simulink model "QuadcopterCompleteModel"  (R2015a)
settings: Solver=ode3  StartTime=0.0  StopTime=20  FixedStep=T_sim  RelTol=1e-5
values from neighbouring files (symbols this model uses):
  A_x = 0.015    [SetupComplete.m]
  A_y = A_x    (= 0.015)    [SetupComplete.m]
  A_z = 0.16    [SetupComplete.m]
  C_x = 1.2    [SetupComplete.m]
  C_y = C_x    (= 1.2)    [SetupComplete.m]
  C_z = 2.2    [SetupComplete.m]
  CG = [0,0,0.02]    [SetupComplete.m]
  I_BAC = diag( [Ix,Iy,Iz])    [SetupComplete.m]
  Initial_Omegas = Omega_hover*ones(4,1)    [Run4Copter.m]
  Initial_Torques = Torque_hover*ones(4,1)    [Run4Copter.m]
  k_quat = 100    [SetupComplete.m]
  l = 0.345    [SetupComplete.m]
  m = 3.51    [SetupComplete.m]
  M_eq = 0.001    [SetupComplete.m]
  R = 0.254    [SetupComplete.m]
  rho = 1.225    [SetupComplete.m]
  Rotation_sign = [ 1,-1,1,-1]    [SetupComplete.m]
  throtle_0 = 0.4    [Run4Copter.m]
undefined symbols (not defined in the file or in its folder): DOWN_0, EAST_0, NORTH_0, P_0, Q_0, R_0, U_0, V_0, W_0
libraries: MCopter x5, simulink_extras x1
settings Model: ExtModeTrigDuration=5000  Creator=alumno4  LastModifiedBy=David
settings SolverCC: PositivePriorityOrder=on
settings DataIOCC: ExternalInput=getinputstruct(op_trim1)  InitialState=getstatestruct(op_trim1)  SignalLoggingSaveFormat=ModelDataLogs
settings OptimizationCC: InlineParams=on  ExpressionDepthLimit=2147483647
settings DebuggingCC: UnderspecifiedInitializationDetection=Classic  MergeDetectMultiDrivingBlocksExec=none  SolverPrmCheckMsg=warning  FcnCallInpInsideContextMsg=UseLocalSettings  StateNameClashWarn=warning
settings RTWCC: SystemTargetFile=quarc_windows.tlc  TemplateMakefile=quarc_default_tmf  Description=QUARC Win32 Target
settings STFCustomTargetCC: TargetLibSuffix=.lib  TargetPreCompLibLocation=C:\PROGRA~2\QUARC\lib\2011a\windows\release  CodeReplacementLibrary=C89/C90 (ANSI)  GenerateSampleERTMain=off  GeneratePreprocessorConditionals=Disable all  ERTCustomFileBanners=off  SupportNonInlinedSFcns=on  SupportVariableSizeSignals=off  MATLABClassNameForMDSCustomization=Simulink.SoftwareTarget.GRTCustomization  CPPClassGenCompliant=on  GRTInterface=on  SystemTargetFile=quarc_windows.tlc
settings GRTTargetCC: TargetPreCompLibLocation=C:\PROGRA~2\QUARC\lib\2011a\windows\release  CodeReplacementLibrary=C89/C90 (ANSI)  ParMdlRefBuildCompliant=off  CompOptLevelCompliant=off  ConcurrentExecutionCompliant=off  CombineOutputUpdateFcns=off  MatFileLogging=off  GRTInterface=on  ExtMode=on  ExtModeMexFile=quarc_comm

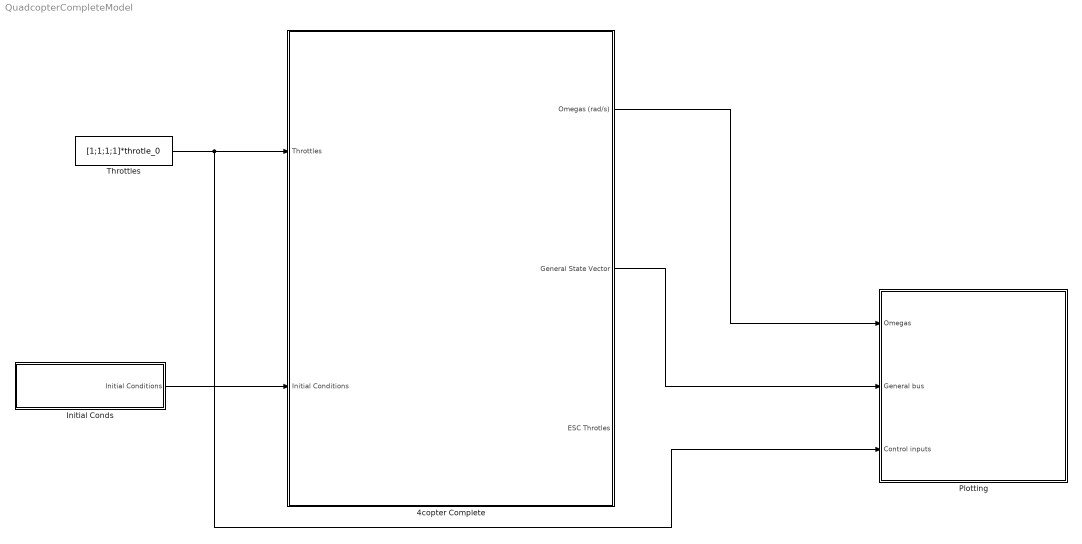
== system QuadcopterCompleteModel ==
  4copter Complete : Subsystem  TreatAsAtomicUnit=on
  Initial Conds : Subsystem  TreatAsAtomicUnit=on
  Plotting : Subsystem
  Throttles : Constant  Value=[1;1;1;1]*throtle_0
  wires:
  Initial Conds/1(Initial Conditions) -> 4copter Complete/2(Initial Conditions)
  Throttles/1 -> Plotting/3(Control inputs), 4copter Complete/1(Throttles)
  4copter Complete/1(Omegas (rad/s)) -> Plotting/1(Omegas)
  4copter Complete/2(General State Vector) -> Plotting/2(General bus)

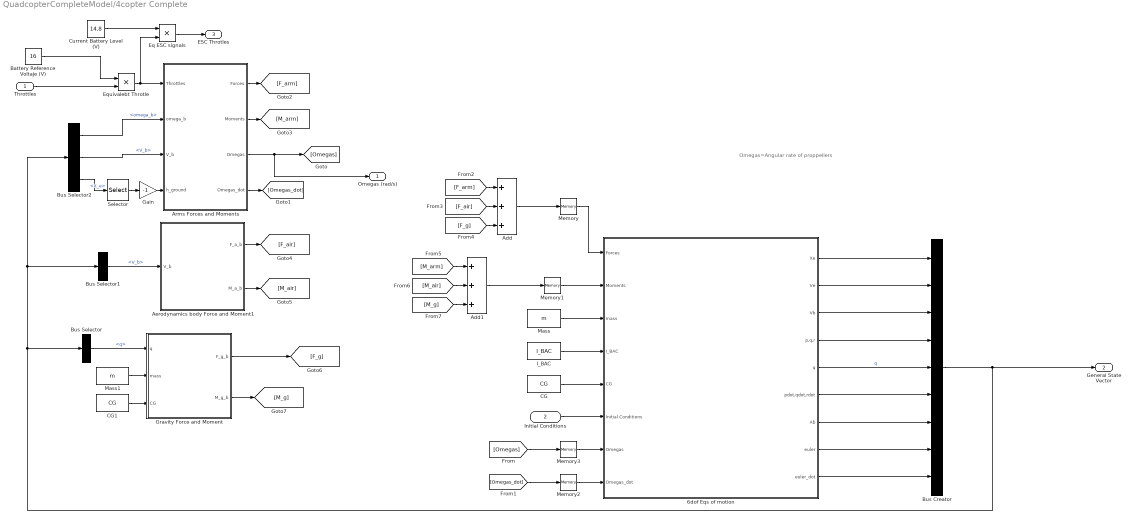
== system QuadcopterCompleteModel/4copter Complete ==
  note: Omegas=Angular rate of proppellers
  Throttles : Inport
  Initial Conditions : Inport  Port=2
  6dof Eqs of motion : Subsystem  TreatAsAtomicUnit=on
  Add : Sum  Inputs=+++
  Add1 : Sum  Inputs=+++
  Aerodynamics body Force and Moment1 : MATLAB Function  TreatAsAtomicUnit=on
  Arms Forces and Moments : Subsystem  TreatAsAtomicUnit=on
  Battery Reference Voltaje (V) : Constant  Value=16
  Bus Creator : BusCreator  Inputs=9
  Bus Selector : BusSelector  OutputSignals=q
  Bus Selector1 : BusSelector  OutputSignals=V_b
  Bus Selector2 : BusSelector  OutputSignals=omega_b,V_b,X_e
  CG : Constant  Value=CG
  CG1 : Constant  Value=CG
  Current Battery Level (V) : Constant  Value=14.8
  Eq ESC signals : Product  Inputs=**
  Equivalebt Throtle : Product  Inputs=**
  Gain : Gain  Gain=-1
  Gravity Force and Moment : MATLAB Function  TreatAsAtomicUnit=on
  I_BAC : Constant  Value=I_BAC
  Mass : Constant  Value=m
  Mass1 : Constant  Value=m
  Memory : Memory  X0=[0,0,0]'
  Memory1 : Memory  X0=[0,0,0]'
  Memory2 : Memory  X0=[0,0,0,0]'
  Memory3 : Memory  X0=Initial_Omegas
  Selector : Selector  InputPortWidth=3  Indices=3
  Omegas (rad/s) : Outport
  General State Vector : Outport  Port=2
  ESC Throtles : Outport  Port=3
  wires:
  Initial Conditions/1 -> 6dof Eqs of motion/6(Initial Conditions)
  6dof Eqs of motion/4(p,q,r) -> Bus Creator/4
  6dof Eqs of motion/3(Vb) -> Bus Creator/3
  6dof Eqs of motion/5(q) -> Bus Creator/5  "q"
  6dof Eqs of motion/2(Ve) -> Bus Creator/2
  6dof Eqs of motion/6(pdot,qdot,rdot) -> Bus Creator/6
  6dof Eqs of motion/1(Xe) -> Bus Creator/1
  6dof Eqs of motion/7(Ab) -> Bus Creator/7
  6dof Eqs of motion/8(euler) -> Bus Creator/8
  6dof Eqs of motion/9(euler_dot) -> Bus Creator/9
  Bus Selector/1 -> Gravity Force and Moment/1(q)  "<q>"
  Mass/1 -> 6dof Eqs of motion/3(mass)
  CG/1 -> 6dof Eqs of motion/5(CG)
  I_BAC/1 -> 6dof Eqs of motion/4(I_BAC)
  Bus Selector1/1 -> Aerodynamics body Force and Moment1/1(V_b)  "<V_b>"
  Bus Selector2/1 -> Arms Forces and Moments/2(omega_b)  "<omega_b>"
  Bus Selector2/2 -> Arms Forces and Moments/3(V_b)  "<V_b>"
  Bus Creator/1 -> Bus Selector1/1, Bus Selector2/1, Bus Selector/1, General State Vector/1
  Mass1/1 -> Gravity Force and Moment/2(mass)
  CG1/1 -> Gravity Force and Moment/3(CG)
  Arms Forces and Moments/3(Omegas) -> Omegas (rad/s)/1, [Omegas]
  Arms Forces and Moments/4(Omegas_dot) -> [Omegas_dot]
  [Omegas] -> Memory3/1
  [Omegas_dot] -> Memory2/1
  Bus Selector2/3 -> Selector/1  "<X_e>"
  Selector/1 -> Gain/1
  Gain/1 -> Arms Forces and Moments/4(h_ground)
  Add/1 -> Memory/1
  Add1/1 -> Memory1/1
  Arms Forces and Moments/1(Forces) -> [F_arm]
  Arms Forces and Moments/2(Moments) -> [M_arm]
  Aerodynamics body Force and Moment1/2(M_a_b) -> [M_air]
  Gravity Force and Moment/1(F_g_b) -> [F_g]
  Gravity Force and Moment/2(M_g_b) -> [M_g]
  [F_arm] -> Add/1
  [F_air] -> Add/2
  [F_g] -> Add/3
  [M_arm] -> Add1/1
  [M_g] -> Add1/3
  [M_air] -> Add1/2
  Memory/1 -> 6dof Eqs of motion/1(Forces)
  Memory1/1 -> 6dof Eqs of motion/2(Moments)
  Memory2/1 -> 6dof Eqs of motion/8(Omegas_dot)
  Memory3/1 -> 6dof Eqs of motion/7(Omegas)
  Equivalebt Throtle/1 -> Eq ESC signals/2, Arms Forces and Moments/1(Throttles)
  Battery Reference Voltaje (V)/1 -> Equivalebt Throtle/1
  Throttles/1 -> Equivalebt Throtle/2
  Eq ESC signals/1 -> ESC Throtles/1
  Current Battery Level (V)/1 -> Eq ESC signals/1
  Aerodynamics body Force and Moment1/1(F_a_b) -> [F_air]

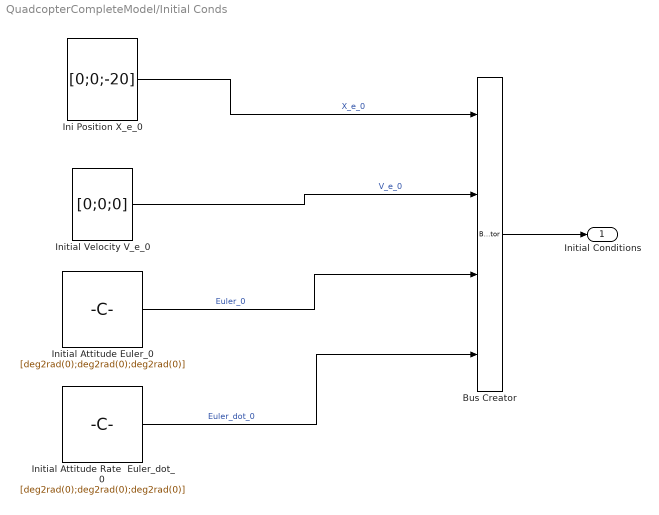
== system QuadcopterCompleteModel/Initial Conds ==
  Bus Creator : BusCreator
  Ini Position X_e_0 : Constant  Value=[0;0;-20]
  Initial Attitude Euler_0 : Constant  Value=[deg2rad(0);deg2rad(0);deg2rad(0)]
  Initial Attitude Rate  Euler_dot_0 : Constant  Value=[deg2rad(0);deg2rad(0);deg2rad(0)]
  Initial Velocity V_e_0 : Constant  Value=[0;0;0]
  Initial Conditions : Outport
  wires:
  Ini Position X_e_0/1 -> Bus Creator/1  "X_e_0"
  Initial Velocity V_e_0/1 -> Bus Creator/2  "V_e_0"
  Initial Attitude Euler_0/1 -> Bus Creator/3  "Euler_0"
  Initial Attitude Rate  Euler_dot_0/1 -> Bus Creator/4  "Euler_dot_0"
  Bus Creator/1 -> Initial Conditions/1

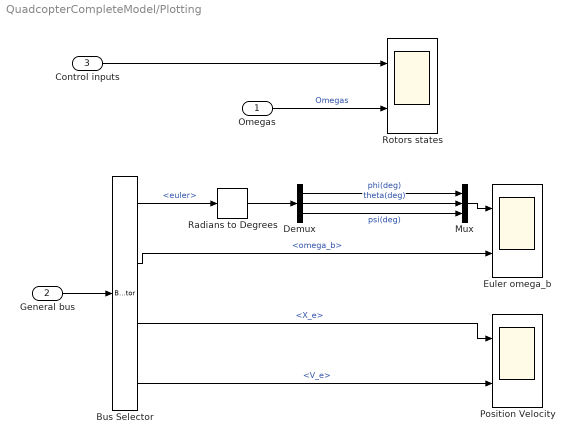
== system QuadcopterCompleteModel/Plotting ==
  Omegas : Inport
  General bus : Inport  Port=2
  Control inputs : Inport  Port=3
  Bus Selector : BusSelector  OutputSignals=euler,omega_b,X_e,V_e
  Demux : Demux  Outputs=3
  Euler omega_b : Scope  NumInputPorts=2
      settings: ShowLegends=on  TimeRange=50  YMin=-45~-0.8  YMax=35~0.7
  Mux : Mux  Inputs=3
  Position Velocity : Scope  NumInputPorts=2
      settings: ShowLegends=on  TimeRange=2  YMin=-20~0  YMax=0~0.8  SaveName=ScopeData8
  Radians to Degrees : simulink_extras/Transformations/Radians to Degrees
  Rotors states : Scope  NumInputPorts=2
      settings: ShowLegends=on  TimeRange=2  YMin=-0.6~640  YMax=1.4~670
  wires:
  General bus/1 -> Bus Selector/1
  Bus Selector/1 -> Radians to Degrees/1  "<euler>"
  Omegas/1 -> Rotors states/2  "Omegas"
  Bus Selector/3 -> Position Velocity/1  "<X_e>"
  Demux/3 -> Mux/3  "psi(deg)"
  Demux/1 -> Mux/1  "phi(deg)"
  Demux/2 -> Mux/2  "theta(deg)"
  Mux/1 -> Euler omega_b/1
  Bus Selector/2 -> Euler omega_b/2  "<omega_b>"
  Control inputs/1 -> Rotors states/1
  Radians to Degrees/1 -> Demux/1
  Bus Selector/4 -> Position Velocity/2  "<V_e>"

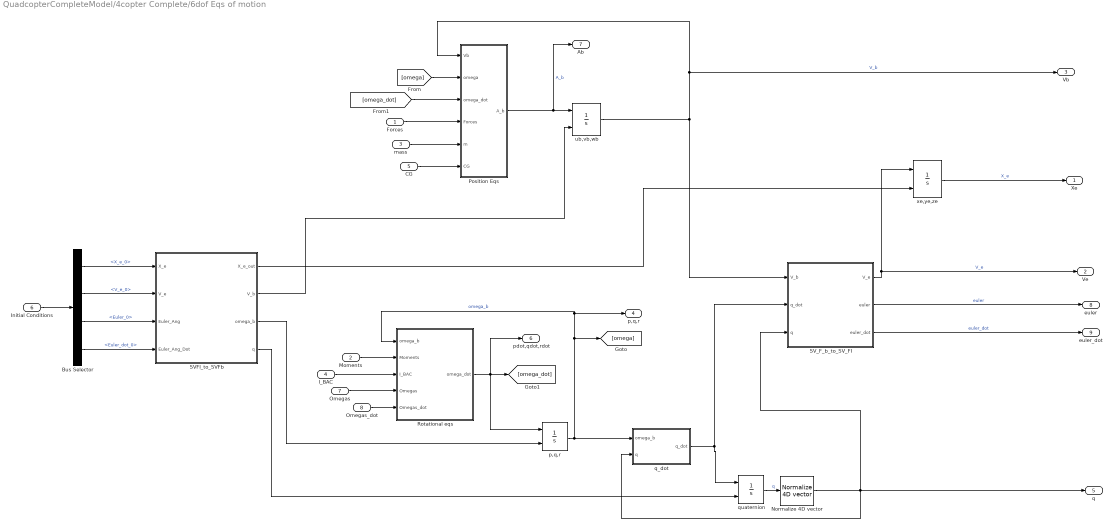
== system QuadcopterCompleteModel/4copter Complete/6dof Eqs of motion ==
  Forces : Inport
  Moments : Inport  Port=2
  mass : Inport  Port=3
  I_BAC : Inport  Port=4
  CG : Inport  Port=5
  Initial Conditions : Inport  Port=6
  Omegas : Inport  Port=7
  Omegas_dot : Inport  Port=8
  Bus Selector : BusSelector  OutputSignals=X_e_0,V_e_0,Euler_0,Euler_dot_0
  Normalize 4D vector : MCopter/Normalize 4D vector
  Position Eqs : MATLAB Function  TreatAsAtomicUnit=on
  Rotational eqs : MATLAB Function  TreatAsAtomicUnit=on
  SVFI_to_SVFb : MATLAB Function  TreatAsAtomicUnit=on
  SV_F_b_to_SV_FI : MATLAB Function  TreatAsAtomicUnit=on
  "p,q,r " : Integrator  InitialConditionSource=external  InitialCondition=[P_0,Q_0,R_0]
  q_dot : Subsystem  TreatAsAtomicUnit=on
  quaternion : Integrator  InitialConditionSource=external  InitialCondition=[P_0,Q_0,R_0]
  ub,vb,wb : Integrator  InitialConditionSource=external  InitialCondition=[U_0,V_0,W_0]
  xe,ye,ze : Integrator  InitialConditionSource=external  InitialCondition=[NORTH_0,EAST_0,-DOWN_0]
  Xe : Outport
  Ve : Outport  Port=2
  Vb : Outport  Port=3
  p,q,r : Outport  Port=4
  q : Outport  Port=5
  pdot,qdot,rdot : Outport  Port=6
  Ab : Outport  Port=7
  euler : Outport  Port=8
  euler_dot : Outport  Port=9
  wires:
  I_BAC/1 -> Rotational eqs/3(I_BAC)
  mass/1 -> Position Eqs/5(m)
  Forces/1 -> Position Eqs/4(Forces)
  xe,ye,ze/1 -> Xe/1  "X_e"
  ub,vb,wb/1 -> Vb/1, Position Eqs/1(Vb), SV_F_b_to_SV_FI/1(V_b)  "V_b"
  SV_F_b_to_SV_FI/1(V_e) -> Ve/1, xe,ye,ze/1  "V_e"
  [omega] -> Position Eqs/2(omega)
  [omega_dot] -> Position Eqs/3(omega_dot)
  Position Eqs/1(A_b) -> Ab/1, ub,vb,wb/1  "A_b"
  CG/1 -> Position Eqs/6(CG)
  Initial Conditions/1 -> Bus Selector/1
  Bus Selector/1 -> SVFI_to_SVFb/1(X_e)  "<X_e_0>"
  Bus Selector/2 -> SVFI_to_SVFb/2(V_e)  "<V_e_0>"
  Bus Selector/3 -> SVFI_to_SVFb/3(Euler_Ang)  "<Euler_0>"
  Bus Selector/4 -> SVFI_to_SVFb/4(Euler_Ang_Dot)  "<Euler_dot_0>"
  SVFI_to_SVFb/2(V_b) -> ub,vb,wb/2
  SVFI_to_SVFb/1(X_e_out) -> xe,ye,ze/2
  SVFI_to_SVFb/3(omega_b) -> "p,q,r "/2
  Rotational eqs/1(omega_dot) -> pdot,qdot,rdot/1, [omega_dot], "p,q,r "/1
  "p,q,r "/1 -> q_dot/1(omega_b), [omega], p,q,r/1, Rotational eqs/1(omega_b)  "omega_b"
  q_dot/1(q_dot) -> quaternion/1, SV_F_b_to_SV_FI/2(q_dot)
  SVFI_to_SVFb/4(q) -> quaternion/2
  quaternion/1 -> Normalize 4D vector/1  "q"
  SV_F_b_to_SV_FI/2(euler) -> euler/1  "euler"
  SV_F_b_to_SV_FI/3(euler_dot) -> euler_dot/1  "euler_dot"
  Moments/1 -> Rotational eqs/2(Moments)
  Omegas/1 -> Rotational eqs/4(Omegas)
  Omegas_dot/1 -> Rotational eqs/5(Omegas_dot)
  Normalize 4D vector/1 -> SV_F_b_to_SV_FI/3(q), q/1, q_dot/2(q)

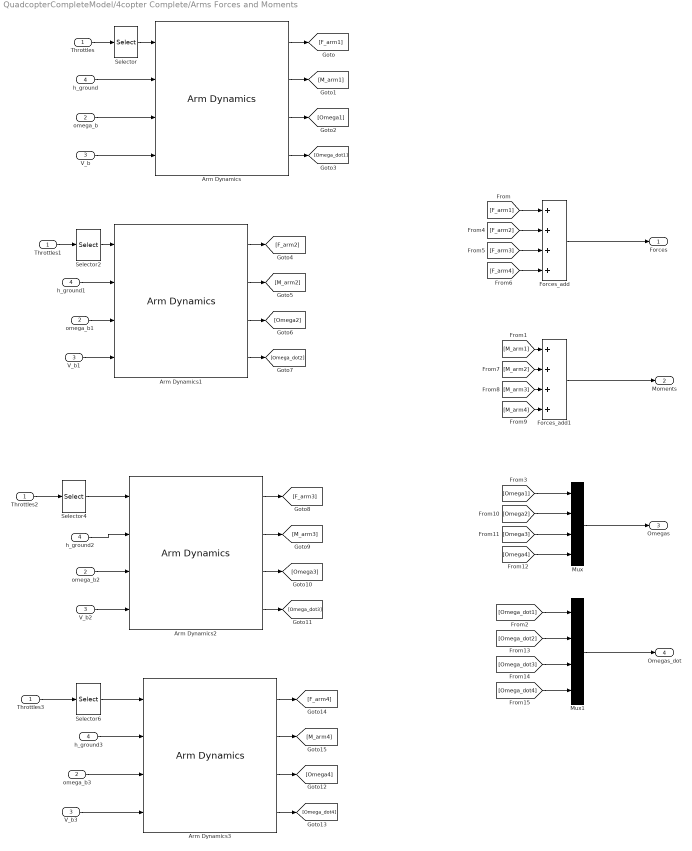
== system QuadcopterCompleteModel/4copter Complete/Arms Forces and Moments ==
  Throttles : Inport
  omega_b : Inport  Port=2
  V_b : Inport  Port=3
  h_ground : Inport  Port=4
  Arm Dynamics : MCopter/Arm Dynamics  Rot_sign=Rotation_sign(1)  arm_num=1  tau=Tau_motors  arm_hub_pos=l*[1;0;0]  J_T=J_T  h=h  Torq_ini=Initial_Torques(1)  Omega_ini=Initial_Omegas(1)
  Arm Dynamics1 : MCopter/Arm Dynamics  Rot_sign=Rotation_sign(2)  arm_num=2  tau=Tau_motors  arm_hub_pos=l*[0;1;0]  J_T=J_T  h=h  Torq_ini=Initial_Torques(2)  Omega_ini=Initial_Omegas(2)
  Arm Dynamics2 : MCopter/Arm Dynamics  Rot_sign=Rotation_sign(3)  arm_num=3  tau=Tau_motors  arm_hub_pos=l*[-1;0;0]  J_T=J_T  h=h  Torq_ini=Initial_Torques(3)  Omega_ini=Initial_Omegas(3)
  Arm Dynamics3 : MCopter/Arm Dynamics  Rot_sign=Rotation_sign(4)  arm_num=4  tau=Tau_motors  arm_hub_pos=l*[0;-1;0]  J_T=J_T  h=h  Torq_ini=Initial_Torques(4)  Omega_ini=Initial_Omegas(4)
  Forces_add : Sum  Inputs=++++
  Forces_add1 : Sum  Inputs=++++
  Mux : Mux
  Mux1 : Mux
  Selector : Selector  InputPortWidth=4  Indices=[1]
  Selector2 : Selector  InputPortWidth=4  Indices=2
  Selector4 : Selector  InputPortWidth=4  Indices=3
  Selector6 : Selector  InputPortWidth=4  Indices=4
  Throttles1 : InportShadow
  Throttles2 : InportShadow
  Throttles3 : InportShadow
  V_b1 : InportShadow  Port=3
  V_b2 : InportShadow  Port=3
  V_b3 : InportShadow  Port=3
  h_ground1 : InportShadow  Port=4
  h_ground2 : InportShadow  Port=4
  h_ground3 : InportShadow  Port=4
  omega_b1 : InportShadow  Port=2
  omega_b2 : InportShadow  Port=2
  omega_b3 : InportShadow  Port=2
  Forces : Outport
  Moments : Outport  Port=2
  Omegas : Outport  Port=3
  Omegas_dot : Outport  Port=4
  wires:
  Throttles/1 -> Selector/1
  Selector/1 -> Arm Dynamics/1
  V_b/1 -> Arm Dynamics/4
  Forces_add/1 -> Forces/1
  Forces_add1/1 -> Moments/1
  Mux/1 -> Omegas/1
  Mux1/1 -> Omegas_dot/1
  h_ground/1 -> Arm Dynamics/2
  Arm Dynamics/1 -> [F_arm1]
  Arm Dynamics/2 -> [M_arm1]
  Arm Dynamics/3 -> [Omega1]
  Arm Dynamics/4 -> [Omega_dot1]
  [F_arm1] -> Forces_add/1
  [M_arm1] -> Forces_add1/1
  [Omega_dot1] -> Mux1/1
  [Omega1] -> Mux/1
  omega_b/1 -> Arm Dynamics/3
  Throttles1/1 -> Selector2/1
  Arm Dynamics1/1 -> [F_arm2]
  Arm Dynamics1/2 -> [M_arm2]
  Arm Dynamics1/3 -> [Omega2]
  Arm Dynamics1/4 -> [Omega_dot2]
  Throttles2/1 -> Selector4/1
  Selector4/1 -> Arm Dynamics2/1
  Arm Dynamics2/1 -> [F_arm3]
  Arm Dynamics2/2 -> [M_arm3]
  Arm Dynamics2/3 -> [Omega3]
  Arm Dynamics2/4 -> [Omega_dot3]
  Throttles3/1 -> Selector6/1
  Selector6/1 -> Arm Dynamics3/1
  Arm Dynamics3/1 -> [F_arm4]
  Arm Dynamics3/2 -> [M_arm4]
  Arm Dynamics3/3 -> [Omega4]
  Arm Dynamics3/4 -> [Omega_dot4]
  [F_arm2] -> Forces_add/2
  [F_arm3] -> Forces_add/3
  [F_arm4] -> Forces_add/4
  [Omega2] -> Mux/2
  [Omega3] -> Mux/3
  [Omega4] -> Mux/4
  [Omega_dot2] -> Mux1/2
  [Omega_dot3] -> Mux1/3
  [Omega_dot4] -> Mux1/4
  [M_arm4] -> Forces_add1/4
  [M_arm3] -> Forces_add1/3
  [M_arm2] -> Forces_add1/2
  Selector2/1 -> Arm Dynamics1/1
  h_ground1/1 -> Arm Dynamics1/2
  omega_b1/1 -> Arm Dynamics1/3
  V_b1/1 -> Arm Dynamics1/4
  omega_b2/1 -> Arm Dynamics2/3
  V_b2/1 -> Arm Dynamics2/4
  h_ground2/1 -> Arm Dynamics2/2
  omega_b3/1 -> Arm Dynamics3/3
  V_b3/1 -> Arm Dynamics3/4
  h_ground3/1 -> Arm Dynamics3/2

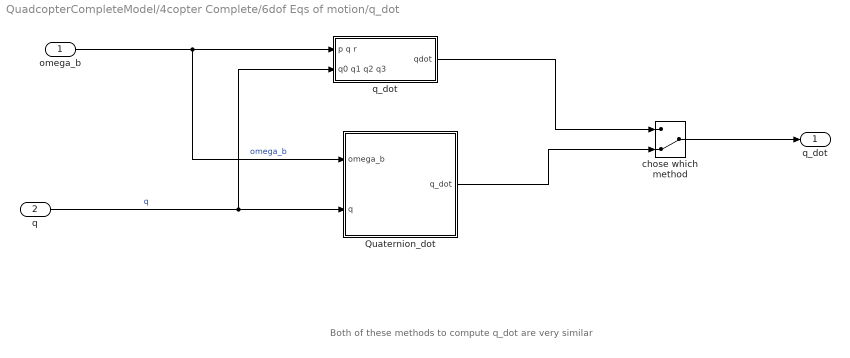
== system QuadcopterCompleteModel/4copter Complete/6dof Eqs of motion/q_dot ==
  note: Both of these methods to compute q_dot are very similar
  omega_b : Inport
  q : Inport  Port=2
  Quaternion_dot : MATLAB Function  TreatAsAtomicUnit=on  VariantControl=Variant
  chose which method : ManualSwitch  CurrentSetting=0
  "q_dot " : Subsystem  TreatAsAtomicUnit=on
  q_dot : Outport
  wires:
  omega_b/1 -> "q_dot "/1(p q r), Quaternion_dot/1(omega_b)  "omega_b"
  q/1 -> "q_dot "/2(q0 q1 q2 q3), Quaternion_dot/2(q)  "q"
  chose which method/1 -> q_dot/1
  "q_dot "/1(qdot) -> chose which method/1
  Quaternion_dot/1(q_dot) -> chose which method/2

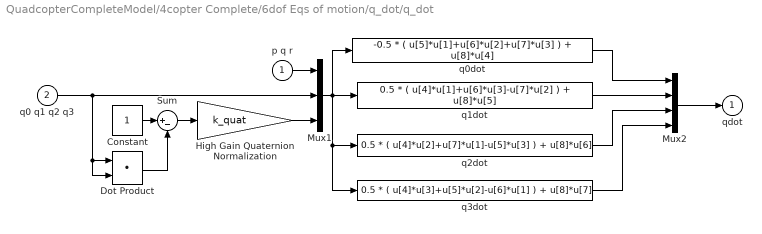
== system QuadcopterCompleteModel/4copter Complete/6dof Eqs of motion/q_dot/q_dot  ==
  p q r : Inport
  q0 q1 q2 q3 : Inport  Port=2
  Constant : Constant
  Dot Product : DotProduct  OutDataTypeStr=Inherit: Inherit via internal rule
  High Gain Quaternion Normalization : Gain  Gain=k_quat  SaturateOnIntegerOverflow=on  OutDataTypeStr=Inherit: Same as input  ParamDataTypeStr=Inherit: Same as input
  Mux1 : Mux  Inputs=[3 4 1]
  Mux2 : Mux
  Sum : Sum  Inputs=|+-  SaturateOnIntegerOverflow=on  InputSameDT=on  OutDataTypeStr=Inherit: Same as first input
  q0dot : Fcn  Expr=-0.5 * ( u[5]*u[1]+u[6]*u[2]+u[7]*u[3] ) + u[8]*u[4]
  q1dot : Fcn  Expr=0.5 * ( u[4]*u[1]+u[6]*u[3]-u[7]*u[2] ) + u[8]*u[5]
  q2dot : Fcn  Expr=0.5 * ( u[4]*u[2]+u[7]*u[1]-u[5]*u[3] ) + u[8]*u[6]
  q3dot : Fcn  Expr=0.5 * ( u[4]*u[3]+u[5]*u[2]-u[6]*u[1] ) + u[8]*u[7]
  qdot : Outport  InitialOutput=0
  wires:
  p q r/1 -> Mux1/1
  Dot Product/1 -> Sum/2
  High Gain Quaternion Normalization/1 -> Mux1/3
  Sum/1 -> High Gain Quaternion Normalization/1
  Constant/1 -> Sum/1
  Mux2/1 -> qdot/1
  q0dot/1 -> Mux2/1
  q1dot/1 -> Mux2/2
  q2dot/1 -> Mux2/3
  Mux1/1 -> q2dot/1, q3dot/1, q0dot/1, q1dot/1
  q3dot/1 -> Mux2/4
  q0 q1 q2 q3/1 -> Dot Product/1, Dot Product/2, Mux1/2

== matlab function QuadcopterCompleteModel/4copter Complete/6dof Eqs of motion/Position Eqs ==
  data: A_b output; Vb input; omega input size=[3,1]; omega_dot input size=[3,1]; Forces input; m input; CG input
function A_b  = PositionEqs(Vb,omega,omega_dot, Forces,m, CG)




A_b =  1/m*( Forces ) - cross(omega,Vb) - cross(omega, cross(omega,CG)) -cross(omega_dot,CG)  ;

== matlab function QuadcopterCompleteModel/4copter Complete/6dof Eqs of motion/Rotational eqs ==
  data: omega_dot output; omega_b input; Moments input; I_BAC input; Omegas input; Omegas_dot input; Rotation_sign parameter; M_eq parameter; R parameter
function omega_dot  = Rotational_Eq(omega_b,Moments, I_BAC,Omegas,Omegas_dot,Rotation_sign,M_eq,R)

omega_dot =  I_BAC\( Moments - cross(omega_b,I_BAC*omega_b)...
    -1/2*M_eq*R^2*[0;0; dot(Omegas_dot,Rotation_sign)] ... % Angular accelerations differences
    - 1/2*M_eq*R^2*[omega_b(2);-omega_b(1);0]*(dot(Omegas,Rotation_sign))  ); % Gyroscopics moments

== matlab function QuadcopterCompleteModel/4copter Complete/6dof Eqs of motion/q_dot/Quaternion_dot ==
  data: omega_b input; q_dot output; q input
function q_dot = Quaternion_dot(omega_b,q)


q_dot = 1/2*HamiltonProduct(q,[0;omega_b]);

== matlab function QuadcopterCompleteModel/4copter Complete/Gravity Force and Moment ==
  data: q input; F_g_b output; M_g_b output; mass input; CG input; g parameter
function [F_g_b,M_g_b]   = Grav_Forces_and_Mom( q,mass,CG, g)

Prod=HamiltonProduct([q(1);-q(2);-q(3);-q(4)],HamiltonProduct([0;0;0;mass*g],[q(1);q(2);q(3);q(4)]) ); % q* . g .q

F_g_b= Prod(2:4);
M_g_b=cross(CG,F_g_b);
end

== matlab function QuadcopterCompleteModel/4copter Complete/Aerodynamics body Force and Moment1 ==
  data: V_b input; F_a_b output; M_a_b output; rho parameter; C_x parameter; C_y parameter; C_z parameter; A_x parameter; A_y parameter; A_z parameter
function [F_a_b,M_a_b]   = Aero_body_Forces_and_Mom( V_b, rho,C_x,C_y,C_z,A_x,A_y,A_z)


F_a_b=-1/2*rho*(norm(V_b)^2)*[C_x*A_x;C_y*A_y;C_z*A_z].*( V_b./(norm(V_b)+eps) );
M_a_b=[0;0;0];
end

== matlab function QuadcopterCompleteModel/4copter Complete/6dof Eqs of motion/SVFI_to_SVFb ==
  data: X_e input; V_e input; X_e_out output; V_b output; omega_b output; Euler_Ang input; Euler_Ang_Dot input; q output
function [X_e_out,V_b, omega_b ,q]=SVFI_to_SVFb(X_e,V_e, Euler_Ang,Euler_Ang_Dot)

xp=V_e(1);
yp=V_e(2);
zp=V_e(3);

phi=Euler_Ang(1);
theta=Euler_Ang(2);
psi=Euler_Ang(3);
phip=Euler_Ang_Dot(1);
thetap=Euler_Ang_Dot(2);
psip=Euler_Ang_Dot(3);

%%
X_e_out=X_e;

q = QuaternionfromEuler(phi,theta,psi); 



HamOut=HamiltonProduct([q(1);-q(2);-q(3);-q(4)],HamiltonProduct([0;xp;yp;zp],[q(1);q(2);q(3);q(4)]) );% q* . v . q
V_b=HamOut(2:4);

omega_b=[phip-psip*sin(theta)  ;
         thetap*cos(phi)+psip*cos(theta)*sin(phi);
            -thetap*sin(phi)+psip*cos(theta)*cos(phi)  ];% Ya que es solo una operacion aislada utilizaremos la ecuaciones con rel trigonometricas
end
function [q]=QuaternionfromEuler(phi,theta,psi)
% options=optimset('MaxFunEvals',3000);
% q=fsolve(@QUATERNIONEULER,[0.6,0.4,0.5,0.4]); % Hay que acertar con los angulos poniendo diferentes valores iniciales del quaternion
%     function F=QUATERNIONEULER(q)
%         F=[ tan(phi)-(2*q(3)*q(4)-2*q(1)*q(2))/(2*q(1)^2+2*q(4)^2-1)  ;
%             sin(-theta)-2*q(2)*q(4)-2*q(1)*q(3);
%             tan(psi)-(2*q(2)*q(3)-2*q(1)*q(4))/(2*q(1)^2+2*q(2)^2-1);
%             q(1)^2+q(2)^2+q(3)^2+q(4)^2-1];
%     end  % Este algoritmo da q* !!!!!

q=[ cos(psi/2)*cos(theta/2)*cos(phi/2)+ sin(psi/2)*sin(theta/2)*sin(phi/2) ;
      cos(psi/2)*cos(theta/2)*sin(phi/2)- sin(psi/2)*sin(theta/2)*cos(phi/2) ;
       cos(psi/2)*sin(theta/2)*cos(phi/2)+ sin(psi/2)*cos(theta/2)*sin(phi/2)   ;
        sin(psi/2)*cos(theta/2)*cos(phi/2)- cos(psi/2)*sin(theta/2)*sin(phi/2)      ]; % Esto nos da q !!!
end

== matlab function QuadcopterCompleteModel/4copter Complete/6dof Eqs of motion/SV_F_b_to_SV_FI ==
  data: V_b input; q_dot input; q input; V_e output; euler output; euler_dot output
function [V_e,euler,euler_dot]   = SV_F_b_to_SV_FI(  V_b, q_dot,q)

xp=V_b(1);
yp=V_b(2);
zp=V_b(3);

%% Velocity and position in Earth Frame   q . v . q*

SolProd=HamiltonProduct([q(1);q(2);q(3);q(4)],HamiltonProduct([0;xp;yp;zp],[q(1);-q(2);-q(3);-q(4)]) );
V_e=SolProd(2:4);

%% Actitud en Angulos de Euler y sus derivadas. 
euler=[0,0,0];
euler(1) = atan2(2*q(3)*q(4)+2*q(1)*q(2),2*q(1)^2+2*q(4)^2-1 ); % phi
euler(2) = -asin( 2*q(2)*q(4)-2*q(1)*q(3) ); %  theta
euler(3) = atan2( 2*q(2)*q(3)+2*q(1)*q(4),2*q(1)^2+2*q(2)^2-1 ); %  psi

euler_dot=[0,0,0]';
euler_dot(1,1) = 2/(1+( (2*q(3)*q(4)+2*q(1)*q(2))/(2*q(1)^2+2*q(4)^2-1)  )^2)*[ -(2*q(1)^2*q(2)+ 4*q(1)*q(3)*q(4)-2*q(2)*q(4)^2+q(2))  ,  q(1)*(2*q(1)^2+2*q(4)^2-1)  ,  q(4)*(2*q(1)^2+2*q(4)^2-1)  ,  -(-2*q(1)^2*q(3) +4*q(1)*q(2)*q(4)+2*q(3)*q(4)^2+q(3) ) ]*q_dot.* 1/(2*q(1)^2+2*q(4)^2-1)^2; % Derivada de phi
euler_dot(2,1) = -2/( sqrt(1-4*(q(2)*q(4)-q(1)*q(3))^2)  )*[-q(3),q(4),-q(1),q(2)]*q_dot;  % Theta prima
euler_dot(3,1) = 2/(1+( (2*q(2)*q(3)+2*q(1)*q(4))/(2*q(1)^2+2*q(2)^2-1)  )^2)*[  -(2*q(1)^2*q(4)+4*q(1)*q(2)*q(3)-2*q(2)^2*q(4)+q(4)  ) , 1/2*(q(3)*(4*q(1)^2-4*q(2)^2-2)-8*q(1)*q(2)*q(4) )  ,  q(2)*(2*q(1)^2+2*q(2)^2-1)  , q(1)*(2*q(1)^2+2*q(2)^2-1) ]*q_dot.*1/(2*q(1)^2+2*q(2)^2-1)^2;  % Psi prima


end
